simulink model "problem8"  (R2020a)
settings: Solver=VariableStepAuto  StartTime=0.0  StopTime=10.0  RelTol=1e-3
settings Model: EnablePacing=on  Creator=INDRAJIT MARATHE  LastModifiedBy=HP

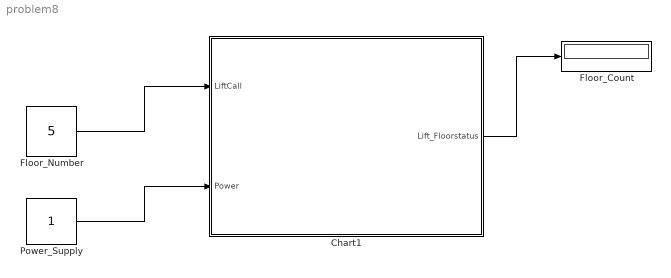
== system problem8 ==
  Chart1 : Stateflow chart  TreatAsAtomicUnit=on
  Floor_Count : Display
  Floor_Number : Constant  Value=5
  Power_Supply : Constant
  wires:
  Power_Supply/1 -> Chart1/2(Power)
  Chart1/1(Lift_Floorstatus) -> Floor_Count/1
  Floor_Number/1 -> Chart1/1(LiftCall)

== stateflow chart problem8/Chart1 ==
  state PowerControl [parallel]
    settings: executionOrder=1
    state Idle
      Lift_Floorstatus=0;
    state Active
    (default) -> Idle : {Lift_Floorstatus=1;}
    Idle -> Active : [Power ==1]
    Active -> Idle : [Power==0]
  state Lift_Status [parallel]
    settings: executionOrder=2
    state Start
    state Down
      du:Lift_Floorstatus=Lift_Floorstatus-1;
    state Up
      du:Lift_Floorstatus=Lift_Floorstatus+1;
    state Wait
    (default) -> Start
    Start -> Down [order 1] : [LiftCall<Lift_Floorstatus]
    Start -> Up [order 2] : [LiftCall>Lift_Floorstatus]
    Down -> Wait : [Lift_Floorstatus==LiftCall]
    Wait -> Start : after(8,sec)
    Up -> Wait : [Lift_Floorstatus==LiftCall]
  data: Lift_Floorstatus output; LiftCall input; Power input
